simulink model "control_system"  (R2020b)
settings: Solver=FixedStepAuto  StartTime=0.0  StopTime=t_sim  FixedStep=Ts  RelTol=1e-2
values from neighbouring files (symbols this model uses):
  Hp = 10    [main_script.m]
  InitPosX = -2.4980e+03    (= -2498)    [main_script.m]
  InitPosY = -650.5503    [main_script.m]
  InitVelX = V0*cosd(InitYaw)    [main_script.m]
  InitVelY = V0*sind(InitYaw)    [main_script.m]
  InitYaw = 21    [main_script.m]
  lr = 1.592    [main_script.m]
  m = 1625    [main_script.m]
  Ts = 0.1    [main_script.m]
  V0 = 25    [main_script.m]
libraries: neural x856, simulink x1, autolibshared x1, drivingscenarioandsensors x1
(part 21 of 40)

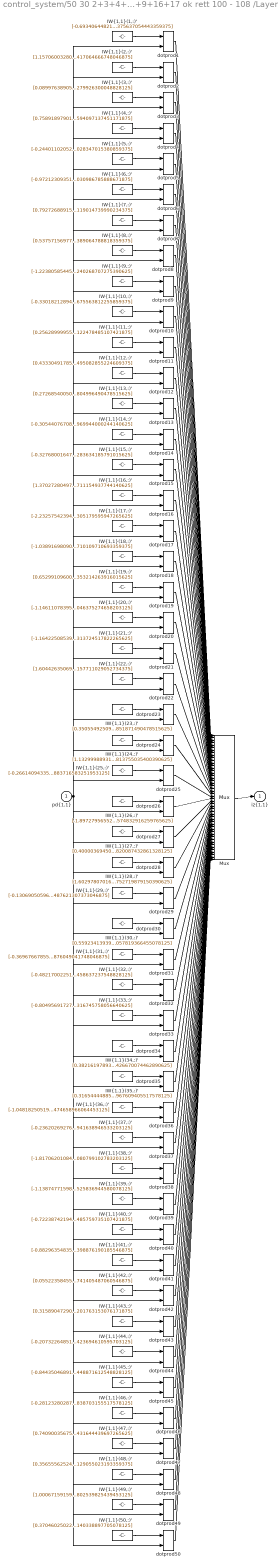
== system control_system/50 30 2+3+4+5+6+7+8+9+16+17 ok rett 100 - 108 /Layer 1/IW{1,1} ==
  "pd{1,1}" : Inport  PortDimensions=9  SampleTime=0.1
      mask Display: e = 0.06;c1 = [120 230 180]/255;c2 = ([120 230 180]+0)/(256+128);c3 = ([120 230 180]+128)/(256+128);patch([0 1 1 0],[0 0 1 1],c1);patch([0 1 1 1-e 1-e 0+e],[0 0 1 1-e 0+e 0+e],c2);patch([0 0 1 1-e 0+e 0+e],[0 1 1 1-e 1-e 0+e],c3);plot([0 1 1 0 0],[0 0 1 1 0]);
  "IW{1,1}(1,:)'" : Constant  Value=[-0.693406448213850001849323234637267887592315673828125;-0.02556518076148506235512058992753736674785614013671875;0.2193186832298505695160173445401596836745738983154296875;1.1520543334356656561823228912544436752796173095703125;-0.40235185759836367136443868730566464364528656005859375;0.90107077061770446402277912056888453662395477294921875;-0.781463922651045361789101661997847259044647216796875;-0.809340341357067227789912067237310111522674560546875;-1.1694920093094791635479623437277041375637054443359375]
      mask Display: e = 0.06;c1 = [120 150 230]/255;c2 = ([120 150 230]+0)/383;c3 = ([120 150 230]+128)/383;patch([0 1 1 0],[0 0 1 1],c1);patch([0 1 1 1-e 1-e 0+e],[0 0 1 1-e 0+e 0+e],c2);patch([0 0 1 1-e 0+e 0+e],[0 1 1 1-e 1-e 0+e],c3);plot([0 1 1 0 0],[0 0 1 1 0]);disp('Weights');
  "IW{1,1}(10,:)'" : Constant  Value=[-0.330182128942806019100686398815014399588108062744140625;0.270379893803715798394904368251445703208446502685546875;-0.97735978725545546996755774671328254044055938720703125;-0.92739473435386254873691314060124568641185760498046875;-0.65365146324644685105198504970758222043514251708984375;2.814218311626336177511120695271529257297515869140625;2.05918257901997403536142883240245282649993896484375;4.88491479731320321633347703027538955211639404296875;-1.173435356109560956383575103245675563812255859375]
      mask Display: e = 0.06;c1 = [120 150 230]/255;c2 = ([120 150 230]+0)/383;c3 = ([120 150 230]+128)/383;patch([0 1 1 0],[0 0 1 1],c1);patch([0 1 1 1-e 1-e 0+e],[0 0 1 1-e 0+e 0+e],c2);patch([0 0 1 1-e 0+e 0+e],[0 1 1 1-e 1-e 0+e],c3);plot([0 1 1 0 0],[0 0 1 1 0]);disp('Weights');
  "IW{1,1}(11,:)'" : Constant  Value=[0.256289999552124891923909899560385383665561676025390625;1.3758001567016198141146787747857160866260528564453125;-0.80612011216949763792172234388999640941619873046875;-0.6585048433570950265902865794487297534942626953125;0.062421786312315645506298977807091432623565196990966796875;0.15111591352368070051426229838398285210132598876953125;-1.301785836379860228362304042093455791473388671875;0.26252656946479202559885379741899669170379638671875;-0.75316510987679929911564613576047122478485107421875]
      mask Display: e = 0.06;c1 = [120 150 230]/255;c2 = ([120 150 230]+0)/383;c3 = ([120 150 230]+128)/383;patch([0 1 1 0],[0 0 1 1],c1);patch([0 1 1 1-e 1-e 0+e],[0 0 1 1-e 0+e 0+e],c2);patch([0 0 1 1-e 0+e 0+e],[0 1 1 1-e 1-e 0+e],c3);plot([0 1 1 0 0],[0 0 1 1 0]);disp('Weights');
  "IW{1,1}(12,:)'" : Constant  Value=[0.43330491785510283353488603097503073513507843017578125;-0.8967160374348315254877661573118530213832855224609375;0.79292956982623585826530643316800706088542938232421875;-0.44560553359943766427164746346534229815006256103515625;0.40491413567924749994375588357797823846340179443359375;-1.8281801022278241219964911579154431819915771484375;-1.794021928142497390723519856692291796207427978515625;1.8148160440597036480170345384976826608180999755859375;0.144981973916790740641857837545103393495082855224609375]
      mask Display: e = 0.06;c1 = [120 150 230]/255;c2 = ([120 150 230]+0)/383;c3 = ([120 150 230]+128)/383;patch([0 1 1 0],[0 0 1 1],c1);patch([0 1 1 1-e 1-e 0+e],[0 0 1 1-e 0+e 0+e],c2);patch([0 0 1 1-e 0+e 0+e],[0 1 1 1-e 1-e 0+e],c3);plot([0 1 1 0 0],[0 0 1 1 0]);disp('Weights');
  "IW{1,1}(13,:)'" : Constant  Value=[0.272685400504414754419002520080539397895336151123046875;0.06475251983479125839071599557428271509706974029541015625;0.0891263580801826271748922181359375827014446258544921875;1.3588154264075875676809346259688027203083038330078125;-0.84834662558519624564468131211469881236553192138671875;-1.7756799833677110456164882634766399860382080078125;-2.108800316675305541735951919690705835819244384765625;2.317421627480893864259314796072430908679962158203125;1.1371762435508954158791539157391525804996490478515625]
      mask Display: e = 0.06;c1 = [120 150 230]/255;c2 = ([120 150 230]+0)/383;c3 = ([120 150 230]+128)/383;patch([0 1 1 0],[0 0 1 1],c1);patch([0 1 1 1-e 1-e 0+e],[0 0 1 1-e 0+e 0+e],c2);patch([0 0 1 1-e 0+e 0+e],[0 1 1 1-e 1-e 0+e],c3);plot([0 1 1 0 0],[0 0 1 1 0]);disp('Weights');
  "IW{1,1}(14,:)'" : Constant  Value=[-0.305440767083966557837726440993719734251499176025390625;1.1031230626814245709965689457021653652191162109375;-0.390168912682526014545913994879811070859432220458984375;1.1610554660892347111911249157856218516826629638671875;-0.37328389762495917114648591450531966984272003173828125;3.2638872617295380251789538306184113025665283203125;0.0203659829001831722827819959320549969561398029327392578125;1.7005610109913560368255502908141352236270904541015625;0.1116923823520036551659728729646303690969944000244140625]
      mask Display: e = 0.06;c1 = [120 150 230]/255;c2 = ([120 150 230]+0)/383;c3 = ([120 150 230]+128)/383;patch([0 1 1 0],[0 0 1 1],c1);patch([0 1 1 1-e 1-e 0+e],[0 0 1 1-e 0+e 0+e],c2);patch([0 0 1 1-e 0+e 0+e],[0 1 1 1-e 1-e 0+e],c3);plot([0 1 1 0 0],[0 0 1 1 0]);disp('Weights');
  "IW{1,1}(15,:)'" : Constant  Value=[-0.32768001647452671409865843088482506573200225830078125;1.172298073364981263466688687913119792938232421875;-0.09920154597840817600751250893154065124690532684326171875;1.4942543874272360415744742567767389118671417236328125;-0.2296467494049061475180906199966557323932647705078125;1.7231626562732567098379377057426609098911285400390625;-0.362349667384589235741287893688422627747058868408203125;1.0058783921240064263002977895666845142841339111328125;0.08797611882380586278973311209483654238283634185791015625]
      mask Display: e = 0.06;c1 = [120 150 230]/255;c2 = ([120 150 230]+0)/383;c3 = ([120 150 230]+128)/383;patch([0 1 1 0],[0 0 1 1],c1);patch([0 1 1 1-e 1-e 0+e],[0 0 1 1-e 0+e 0+e],c2);patch([0 0 1 1-e 0+e 0+e],[0 1 1 1-e 1-e 0+e],c3);plot([0 1 1 0 0],[0 0 1 1 0]);disp('Weights');
  "IW{1,1}(16,:)'" : Constant  Value=[1.37027280497960735061724335537292063236236572265625;0.159288578325931406975968229744466952979564666748046875;1.281773545555778159865667475969530642032623291015625;0.627168919722477458122966709197498857975006103515625;0.53591714582890348506083455504267476499080657958984375;-3.229531631920237177979515763581730425357818603515625;-0.69317652394062323484291709974058903753757476806640625;-2.173242526392685558533912626444362103939056396484375;-0.63066588600048378854268094073631800711154937744140625]
      mask Display: e = 0.06;c1 = [120 150 230]/255;c2 = ([120 150 230]+0)/383;c3 = ([120 150 230]+128)/383;patch([0 1 1 0],[0 0 1 1],c1);patch([0 1 1 1-e 1-e 0+e],[0 0 1 1-e 0+e 0+e],c2);patch([0 0 1 1-e 0+e 0+e],[0 1 1 1-e 1-e 0+e],c3);plot([0 1 1 0 0],[0 0 1 1 0]);disp('Weights');
  "IW{1,1}(17,:)'" : Constant  Value=[-2.232575423946769888061680831015110015869140625;-0.1829004396172365376482815690906136296689510345458984375;1.2677494346707975925170330810942687094211578369140625;-0.87503780474532266708820316125638782978057861328125;0.807021408287351249555285903625190258026123046875;0.23988792042748574573352016159333288669586181640625;1.62198306035521699897117287036962807178497314453125;-0.695423451580790441539647872559726238250732421875;-0.82653776048596316883276813314296305179595947265625]
      mask Display: e = 0.06;c1 = [120 150 230]/255;c2 = ([120 150 230]+0)/383;c3 = ([120 150 230]+128)/383;patch([0 1 1 0],[0 0 1 1],c1);patch([0 1 1 1-e 1-e 0+e],[0 0 1 1-e 0+e 0+e],c2);patch([0 0 1 1-e 0+e 0+e],[0 1 1 1-e 1-e 0+e],c3);plot([0 1 1 0 0],[0 0 1 1 0]);disp('Weights');
  "IW{1,1}(18,:)'" : Constant  Value=[-1.0389169809062208660321857678354717791080474853515625;-1.4630196868647835639620780057157389819622039794921875;0.99642406399851235487830081183346919715404510498046875;-1.170179726715411927528975866152904927730560302734375;-0.51561709388959309219302440396859310567378997802734375;-0.75058668503490622025964285057852976024150848388671875;-0.41577361564194215137746368782245554029941558837890625;0.77508037001214524774894698566640727221965789794921875;-0.748086589386244948940429821959696710109710693359375]
      mask Display: e = 0.06;c1 = [120 150 230]/255;c2 = ([120 150 230]+0)/383;c3 = ([120 150 230]+128)/383;patch([0 1 1 0],[0 0 1 1],c1);patch([0 1 1 1-e 1-e 0+e],[0 0 1 1-e 0+e 0+e],c2);patch([0 0 1 1-e 0+e 0+e],[0 1 1 1-e 1-e 0+e],c3);plot([0 1 1 0 0],[0 0 1 1 0]);disp('Weights');
  "IW{1,1}(19,:)'" : Constant  Value=[0.65299109600750693260806656326167285442352294921875;0.7753435649205380197912518269731663167476654052734375;1.0415876039493869864571706784772686660289764404296875;-0.65848787255995333556057858004351146519184112548828125;1.2322117642516641211614114581607282161712646484375;0.274341649489681593809820014939759857952594757080078125;0.58124655016228865545002690851106308400630950927734375;0.9466010499085590890189223500783555209636688232421875;-0.08066011985930966743385539530208916403353214263916015625]
      mask Display: e = 0.06;c1 = [120 150 230]/255;c2 = ([120 150 230]+0)/383;c3 = ([120 150 230]+128)/383;patch([0 1 1 0],[0 0 1 1],c1);patch([0 1 1 1-e 1-e 0+e],[0 0 1 1-e 0+e 0+e],c2);patch([0 0 1 1-e 0+e 0+e],[0 1 1 1-e 1-e 0+e],c3);plot([0 1 1 0 0],[0 0 1 1 0]);disp('Weights');
  "IW{1,1}(2,:)'" : Constant  Value=[1.1570600328072238038856767161632888019084930419921875;1.903733690245744458735543958027847111225128173828125;-0.389863627068089024785280116702779196202754974365234375;1.746257178047623259686815799796022474765777587890625;0.00989143632890131241364173320107511244714260101318359375;2.7315874512668614215726847760379314422607421875;0.538870059530276446224661412998102605342864990234375;-4.29457801509744996337758493609726428985595703125;1.900650844106816617085087273153476417064666748046875]
      mask Display: e = 0.06;c1 = [120 150 230]/255;c2 = ([120 150 230]+0)/383;c3 = ([120 150 230]+128)/383;patch([0 1 1 0],[0 0 1 1],c1);patch([0 1 1 1-e 1-e 0+e],[0 0 1 1-e 0+e 0+e],c2);patch([0 0 1 1-e 0+e 0+e],[0 1 1 1-e 1-e 0+e],c3);plot([0 1 1 0 0],[0 0 1 1 0]);disp('Weights');
  "IW{1,1}(20,:)'" : Constant  Value=[-1.14611078395096210869041897240094840526580810546875;0.86858056570071473512228976687765680253505706787109375;-1.58842280534746738140938759897835552692413330078125;-0.69376786411447655122941569061367772519588470458984375;0.94198070731023431090278563715401105582714080810546875;-0.94930693977512781156491428191657178103923797607421875;1.1886668013198040672051547517185099422931671142578125;2.44320512274560552867797014187090098857879638671875;0.5842324962664815490853698065620847046375274658203125]
      mask Display: e = 0.06;c1 = [120 150 230]/255;c2 = ([120 150 230]+0)/383;c3 = ([120 150 230]+128)/383;patch([0 1 1 0],[0 0 1 1],c1);patch([0 1 1 1-e 1-e 0+e],[0 0 1 1-e 0+e 0+e],c2);patch([0 0 1 1-e 0+e 0+e],[0 1 1 1-e 1-e 0+e],c3);plot([0 1 1 0 0],[0 0 1 1 0]);disp('Weights');
  "IW{1,1}(21,:)'" : Constant  Value=[-1.1642250853925999454219208928407169878482818603515625;-0.5504932807784437276410471895360387861728668212890625;-1.6869414057329326084300191723741590976715087890625;-0.0028722543247330510791937019376973694306798279285430908203125;0.19023363022934602906133250144193880259990692138671875;-1.20570399485861035060452195466496050357818603515625;-0.1577300337552645093097680728533305227756500244140625;0.2327125275973849494182132957575959153473377227783203125;0.64502475045348950377643859610543586313724517822265625]
      mask Display: e = 0.06;c1 = [120 150 230]/255;c2 = ([120 150 230]+0)/383;c3 = ([120 150 230]+128)/383;patch([0 1 1 0],[0 0 1 1],c1);patch([0 1 1 1-e 1-e 0+e],[0 0 1 1-e 0+e 0+e],c2);patch([0 0 1 1-e 0+e 0+e],[0 1 1 1-e 1-e 0+e],c3);plot([0 1 1 0 0],[0 0 1 1 0]);disp('Weights');
  "IW{1,1}(22,:)'" : Constant  Value=[1.6044263506907328054040817733039148151874542236328125;1.3319671089723590373665729202912189066410064697265625;-1.0851131040152262041686981319799087941646575927734375;2.1355962975134108461361392983235418796539306640625;0.52286735422735119982462492771446704864501953125;-1.645841449463056438418107063625939190387725830078125;1.6714988511291586359419625296141020953655242919921875;-0.1418426114294394080328487461883923970162868499755859375;-1.338735324179674446298804468824528157711029052734375]
      mask Display: e = 0.06;c1 = [120 150 230]/255;c2 = ([120 150 230]+0)/383;c3 = ([120 150 230]+128)/383;patch([0 1 1 0],[0 0 1 1],c1);patch([0 1 1 1-e 1-e 0+e],[0 0 1 1-e 0+e 0+e],c2);patch([0 0 1 1-e 0+e 0+e],[0 1 1 1-e 1-e 0+e],c3);plot([0 1 1 0 0],[0 0 1 1 0]);disp('Weights');
  "IW{1,1}(23,:)'" : Constant  Value=[0.350554925097944225509394300388521514832973480224609375;-1.0931491474881587233625168664730153977870941162109375;0.4203166172719525750522961971000768244266510009765625;-1.394127712399904073237166812759824097156524658203125;-1.3990696404685694087532965568243525922298431396484375;-0.236876967776770808171704629785381257534027099609375;-0.305940597094979171988171628981945104897022247314453125;-0.216334751492993360155736581873497925698757171630859375;0.81177408117963223421753582442761398851871490478515625]
      mask Display: e = 0.06;c1 = [120 150 230]/255;c2 = ([120 150 230]+0)/383;c3 = ([120 150 230]+128)/383;patch([0 1 1 0],[0 0 1 1],c1);patch([0 1 1 1-e 1-e 0+e],[0 0 1 1-e 0+e 0+e],c2);patch([0 0 1 1-e 0+e 0+e],[0 1 1 1-e 1-e 0+e],c3);plot([0 1 1 0 0],[0 0 1 1 0]);disp('Weights');
  "IW{1,1}(24,:)'" : Constant  Value=[1.1329998893150687866437920092721469700336456298828125;-1.4321153177865941774626890037325210869312286376953125;2.591323690879150820620679951389320194721221923828125;1.0806065027108360254715080372989177703857421875;-1.867832138149747578381720813922584056854248046875;1.9590467197986949354771013531717471778392791748046875;1.00821489655478568892021939973346889019012451171875;-0.7955102958743938135199869066127575933933258056640625;-0.59861999316104397284021843006485141813755035400390625]
      mask Display: e = 0.06;c1 = [120 150 230]/255;c2 = ([120 150 230]+0)/383;c3 = ([120 150 230]+128)/383;patch([0 1 1 0],[0 0 1 1],c1);patch([0 1 1 1-e 1-e 0+e],[0 0 1 1-e 0+e 0+e],c2);patch([0 0 1 1-e 0+e 0+e],[0 1 1 1-e 1-e 0+e],c3);plot([0 1 1 0 0],[0 0 1 1 0]);disp('Weights');
  "IW{1,1}(25,:)'" : Constant  Value=[-0.266140943359271575641145091140060685575008392333984375;0.93128971553801409566375468784826807677745819091796875;-0.763023833714053356658268967294134199619293212890625;-1.1174471698171324351989142087404616177082061767578125;0.86052416309833967833498036270611919462680816650390625;1.36946534724734902965792571194469928741455078125;-0.08714593803625887702413166380210896022617816925048828125;0.7130613830161605104507316355011425912380218505859375;0.01361678574539722415270848188129093614406883716583251953125]
      mask Display: e = 0.06;c1 = [120 150 230]/255;c2 = ([120 150 230]+0)/383;c3 = ([120 150 230]+128)/383;patch([0 1 1 0],[0 0 1 1],c1);patch([0 1 1 1-e 1-e 0+e],[0 0 1 1-e 0+e 0+e],c2);patch([0 0 1 1-e 0+e 0+e],[0 1 1 1-e 1-e 0+e],c3);plot([0 1 1 0 0],[0 0 1 1 0]);disp('Weights');
  "IW{1,1}(26,:)'" : Constant  Value=[-1.89727956552465304440602267277427017688751220703125;1.2876139672237514322006290967692621052265167236328125;0.83258954146781138927480014899629168212413787841796875;-2.91139210909474410726716087083332240581512451171875;0.32359731118500378865832090014009736478328704833984375;0.384597586722556117333482461617677472531795501708984375;-0.868477310397982815715067772543989121913909912109375;-0.5317092104185012768624574164277873933315277099609375;1.2926350037718228325189784300164319574832916259765625]
      mask Display: e = 0.06;c1 = [120 150 230]/255;c2 = ([120 150 230]+0)/383;c3 = ([120 150 230]+128)/383;patch([0 1 1 0],[0 0 1 1],c1);patch([0 1 1 1-e 1-e 0+e],[0 0 1 1-e 0+e 0+e],c2);patch([0 0 1 1-e 0+e 0+e],[0 1 1 1-e 1-e 0+e],c3);plot([0 1 1 0 0],[0 0 1 1 0]);disp('Weights');
  "IW{1,1}(27,:)'" : Constant  Value=[0.400003694501827322671516640184563584625720977783203125;-0.85527108082092018204178884843713603913784027099609375;1.4010061502814747935730110839358530938625335693359375;-1.4806639264167633651680944240069948136806488037109375;-0.72477438149454076476985164845245890319347381591796875;1.93831254159486388033428738708607852458953857421875;0.310800466532213548465080066307564266026020050048828125;-2.841585827968680089128383770002983510494232177734375;1.3646232279807606335708669575979001820087432861328125]
      mask Display: e = 0.06;c1 = [120 150 230]/255;c2 = ([120 150 230]+0)/383;c3 = ([120 150 230]+128)/383;patch([0 1 1 0],[0 0 1 1],c1);patch([0 1 1 1-e 1-e 0+e],[0 0 1 1-e 0+e 0+e],c2);patch([0 0 1 1-e 0+e 0+e],[0 1 1 1-e 1-e 0+e],c3);plot([0 1 1 0 0],[0 0 1 1 0]);disp('Weights');
  "IW{1,1}(28,:)'" : Constant  Value=[1.602978070162198065418124315328896045684814453125;-0.3426681801413840045000824829912744462490081787109375;1.529770685331715895927118253894150257110595703125;1.1716836187309633832143163090222515165805816650390625;0.046185804249316120273505248405854217708110809326171875;-0.75021965501111054219762763750622980296611785888671875;1.074021043023239752045583372819237411022186279296875;0.8185220590198494239331239441526122391223907470703125;0.0956170049154911050326433041846030391752719879150390625]
      mask Display: e = 0.06;c1 = [120 150 230]/255;c2 = ([120 150 230]+0)/383;c3 = ([120 150 230]+128)/383;patch([0 1 1 0],[0 0 1 1],c1);patch([0 1 1 1-e 1-e 0+e],[0 0 1 1-e 0+e 0+e],c2);patch([0 0 1 1-e 0+e 0+e],[0 1 1 1-e 1-e 0+e],c3);plot([0 1 1 0 0],[0 0 1 1 0]);disp('Weights');
  "IW{1,1}(29,:)'" : Constant  Value=[-0.1306905059673156010990879849487100727856159210205078125;-0.7876508797924930416201050320523791015148162841796875;-0.51317475975367499163581896937103010714054107666015625;-0.1457425730357558568694997802595025859773159027099609375;-0.70171443760436857939311039444874040782451629638671875;1.27527189707526122930403289501555263996124267578125;0.8890613846162340738743523615994490683078765869140625;0.3216145672896235652160612517036497592926025390625;-1.008127048696333627475496541592292487621307373046875]
      mask Display: e = 0.06;c1 = [120 150 230]/255;c2 = ([120 150 230]+0)/383;c3 = ([120 150 230]+128)/383;patch([0 1 1 0],[0 0 1 1],c1);patch([0 1 1 1-e 1-e 0+e],[0 0 1 1-e 0+e 0+e],c2);patch([0 0 1 1-e 0+e 0+e],[0 1 1 1-e 1-e 0+e],c3);plot([0 1 1 0 0],[0 0 1 1 0]);disp('Weights');
  "IW{1,1}(3,:)'" : Constant  Value=[0.08997638905276246490405611666574259288609027862548828125;0.80681741283027574862529718302539549767971038818359375;0.2250171821611615385894111796005745418369770050048828125;-0.50944131721464402939858473473577760159969329833984375;0.2000247490916989001608072840099339373409748077392578125;1.20314470992705491170227105612866580486297607421875;1.4027922012298004172947685219696722924709320068359375;0.8756386789487733413039904917241074144840240478515625;0.007739900862407400779219290853916390915401279926300048828125]
      mask Display: e = 0.06;c1 = [120 150 230]/255;c2 = ([120 150 230]+0)/383;c3 = ([120 150 230]+128)/383;patch([0 1 1 0],[0 0 1 1],c1);patch([0 1 1 1-e 1-e 0+e],[0 0 1 1-e 0+e 0+e],c2);patch([0 0 1 1-e 0+e 0+e],[0 1 1 1-e 1-e 0+e],c3);plot([0 1 1 0 0],[0 0 1 1 0]);disp('Weights');
  "IW{1,1}(30,:)'" : Constant  Value=[0.55923413939413391116062257424346171319484710693359375;-0.276142396858805538872871920830220915377140045166015625;-0.841140637081708941735769258229993283748626708984375;-1.2799808287890843683243247141945175826549530029296875;0.1619096371925195787522255841395235620439052581787109375;-0.031011122222041880014398174125744844786822795867919921875;-0.67759415806670475479478454872150905430316925048828125;1.1300688296323215809024986810982227325439453125;1.673317340979104006493116685305722057819366455078125]
      mask Display: e = 0.06;c1 = [120 150 230]/255;c2 = ([120 150 230]+0)/383;c3 = ([120 150 230]+128)/383;patch([0 1 1 0],[0 0 1 1],c1);patch([0 1 1 1-e 1-e 0+e],[0 0 1 1-e 0+e 0+e],c2);patch([0 0 1 1-e 0+e 0+e],[0 1 1 1-e 1-e 0+e],c3);plot([0 1 1 0 0],[0 0 1 1 0]);disp('Weights');
  "IW{1,1}(31,:)'" : Constant  Value=[-0.369676678559802074364171176057425327599048614501953125;-0.58159156486953322851007897043018601834774017333984375;1.0786932187140381156353896585642360150814056396484375;0.637537765261984024078856236883439123630523681640625;0.7410181941734403920918339281342923641204833984375;-2.32287606270722779555626402725465595722198486328125;-0.48709727099964605923076987892272882163524627685546875;2.050543368761421181289961168658919632434844970703125;0.48267963789397494434041391286882571876049041748046875]
      mask Display: e = 0.06;c1 = [120 150 230]/255;c2 = ([120 150 230]+0)/383;c3 = ([120 150 230]+128)/383;patch([0 1 1 0],[0 0 1 1],c1);patch([0 1 1 1-e 1-e 0+e],[0 0 1 1-e 0+e 0+e],c2);patch([0 0 1 1-e 0+e 0+e],[0 1 1 1-e 1-e 0+e],c3);plot([0 1 1 0 0],[0 0 1 1 0]);disp('Weights');
  "IW{1,1}(32,:)'" : Constant  Value=[-0.482170022514028573379363251660834066569805145263671875;0.96009191106100166823722474873648025095462799072265625;-0.911853201103436372676469545694999396800994873046875;0.08528072811694854815645072676488780416548252105712890625;1.164210642311785282032587929279543459415435791015625;0.91960001333729401995498164978926070034503936767578125;0.65569530552422905511633643982349894940853118896484375;-1.0546061852062618147130024226498790085315704345703125;-0.63904426441919170986949438884039409458637237548828125]
      mask Display: e = 0.06;c1 = [120 150 230]/255;c2 = ([120 150 230]+0)/383;c3 = ([120 150 230]+128)/383;patch([0 1 1 0],[0 0 1 1],c1);patch([0 1 1 1-e 1-e 0+e],[0 0 1 1-e 0+e 0+e],c2);patch([0 0 1 1-e 0+e 0+e],[0 1 1 1-e 1-e 0+e],c3);plot([0 1 1 0 0],[0 0 1 1 0]);disp('Weights');
  "IW{1,1}(33,:)'" : Constant  Value=[-0.80495691727967433326540458438103087246417999267578125;0.6411180503735127711451013965415768325328826904296875;-1.2023286220364719500963701648288406431674957275390625;-1.599120401012341208257794278324581682682037353515625;-0.0953775174016849580649335393900400958955287933349609375;1.2326435111067846062127273398800753057003021240234375;0.042770745663714880568928577986298478208482265472412109375;1.766417956869078320636390344589017331600189208984375;-0.358630123165513570171469837077893316745758056640625]
      mask Display: e = 0.06;c1 = [120 150 230]/255;c2 = ([120 150 230]+0)/383;c3 = ([120 150 230]+128)/383;patch([0 1 1 0],[0 0 1 1],c1);patch([0 1 1 1-e 1-e 0+e],[0 0 1 1-e 0+e 0+e],c2);patch([0 0 1 1-e 0+e 0+e],[0 1 1 1-e 1-e 0+e],c3);plot([0 1 1 0 0],[0 0 1 1 0]);disp('Weights');
  "IW{1,1}(34,:)'" : Constant  Value=[0.382161978935705970439329348664614371955394744873046875;-0.76302057400596179359553161702933721244335174560546875;0.298250016106143822636198592590517364442348480224609375;-0.70487538233506652485260701723746024072170257568359375;0.0279956842207948232437164648445104830898344516754150390625;-0.68521612708078549758283770643174648284912109375;-0.418788213989499558120854771914309822022914886474609375;-2.727281390156304663463515680632553994655609130859375;-1.277907013729996155149137848638929426670074462890625]
      mask Display: e = 0.06;c1 = [120 150 230]/255;c2 = ([120 150 230]+0)/383;c3 = ([120 150 230]+128)/383;patch([0 1 1 0],[0 0 1 1],c1);patch([0 1 1 1-e 1-e 0+e],[0 0 1 1-e 0+e 0+e],c2);patch([0 0 1 1-e 0+e 0+e],[0 1 1 1-e 1-e 0+e],c3);plot([0 1 1 0 0],[0 0 1 1 0]);disp('Weights');
  "IW{1,1}(35,:)'" : Constant  Value=[0.316544448857396798491237177586299367249011993408203125;0.6155314425673754641366031137295067310333251953125;0.1415964825864601817073662459733895957469940185546875;1.3954169536738867396508112506126053631305694580078125;0.24249578330329757402950008327024988830089569091796875;-1.79231644266071210580548722646199166774749755859375;0.13028961116798576380659824280883185565471649169921875;-0.343855544436020454934777035305160097777843475341796875;-0.75040981724793376361759555948083288967609405517578125]
      mask Display: e = 0.06;c1 = [120 150 230]/255;c2 = ([120 150 230]+0)/383;c3 = ([120 150 230]+128)/383;patch([0 1 1 0],[0 0 1 1],c1);patch([0 1 1 1-e 1-e 0+e],[0 0 1 1-e 0+e 0+e],c2);patch([0 0 1 1-e 0+e 0+e],[0 1 1 1-e 1-e 0+e],c3);plot([0 1 1 0 0],[0 0 1 1 0]);disp('Weights');
  "IW{1,1}(36,:)'" : Constant  Value=[-1.048182505198408609459193030488677322864532470703125;0.5151532139605734528231550939381122589111328125;-2.32440222618064584736430333578027784824371337890625;-0.9589975404242412349020696638035587966442108154296875;-1.161839122224388010096163270645774900913238525390625;-1.8480403874410573639153199110296554863452911376953125;-0.468092609921334001921167100590537302196025848388671875;-2.588322666240973735085617590812034904956817626953125;-0.0293675915841758172764031087353941984474658966064453125]
      mask Display: e = 0.06;c1 = [120 150 230]/255;c2 = ([120 150 230]+0)/383;c3 = ([120 150 230]+128)/383;patch([0 1 1 0],[0 0 1 1],c1);patch([0 1 1 1-e 1-e 0+e],[0 0 1 1-e 0+e 0+e],c2);patch([0 0 1 1-e 0+e 0+e],[0 1 1 1-e 1-e 0+e],c3);plot([0 1 1 0 0],[0 0 1 1 0]);disp('Weights');
  "IW{1,1}(37,:)'" : Constant  Value=[-0.2362026927647044860503200425227987580001354217529296875;-0.78218715596495591579895290124113671481609344482421875;0.8565351137683296922631370762246660888195037841796875;1.4776102515902180822848777097533456981182098388671875;0.453191929204543264564364335456048138439655303955078125;-0.1195925461842739512263733558938838541507720947265625;-0.70882313381148553954602675730711780488491058349609375;-0.480949892098079201385729675166658125817775726318359375;1.5768117638188112739072721524280495941638946533203125]
      mask Display: e = 0.06;c1 = [120 150 230]/255;c2 = ([120 150 230]+0)/383;c3 = ([120 150 230]+128)/383;patch([0 1 1 0],[0 0 1 1],c1);patch([0 1 1 1-e 1-e 0+e],[0 0 1 1-e 0+e 0+e],c2);patch([0 0 1 1-e 0+e 0+e],[0 1 1 1-e 1-e 0+e],c3);plot([0 1 1 0 0],[0 0 1 1 0]);disp('Weights');
  "IW{1,1}(38,:)'" : Constant  Value=[-1.8170620108458077623936333111487329006195068359375;-0.836309493935304626432980512618087232112884521484375;0.347037295405833778882964679723954759538173675537109375;-1.1257424830385394098897222647792659699916839599609375;-1.5102367218942529536462870964896865189075469970703125;-1.16258945977454342113333041197620332241058349609375;0.040529601691721740819307484571254462935030460357666015625;-1.762905379354144930204029151354916393756866455078125;1.369967279907751578349461851757951080799102783203125]
      mask Display: e = 0.06;c1 = [120 150 230]/255;c2 = ([120 150 230]+0)/383;c3 = ([120 150 230]+128)/383;patch([0 1 1 0],[0 0 1 1],c1);patch([0 1 1 1-e 1-e 0+e],[0 0 1 1-e 0+e 0+e],c2);patch([0 0 1 1-e 0+e 0+e],[0 1 1 1-e 1-e 0+e],c3);plot([0 1 1 0 0],[0 0 1 1 0]);disp('Weights');
  "IW{1,1}(39,:)'" : Constant  Value=[-1.1387477159820329486450418698950670659542083740234375;0.12329538400851185186990477404833654873073101043701171875;-1.2901694683843327737804429489187896251678466796875;0.482497177772101382142722059143125079572200775146484375;-0.46053829469796248030633023518021218478679656982421875;0.8066115310647157254919648039503954350948333740234375;0.362412929683291640259312771377153694629669189453125;-0.3922292711960551070404790152679197490215301513671875;-0.9901181825802745084530442909453995525836944580078125]
      mask Display: e = 0.06;c1 = [120 150 230]/255;c2 = ([120 150 230]+0)/383;c3 = ([120 150 230]+128)/383;patch([0 1 1 0],[0 0 1 1],c1);patch([0 1 1 1-e 1-e 0+e],[0 0 1 1-e 0+e 0+e],c2);patch([0 0 1 1-e 0+e 0+e],[0 1 1 1-e 1-e 0+e],c3);plot([0 1 1 0 0],[0 0 1 1 0]);disp('Weights');
  "IW{1,1}(4,:)'" : Constant  Value=[0.75891897901968963235930232258397154510021209716796875;1.0908727108738067723692211075103841722011566162109375;0.175572791832671881717686801493982784450054168701171875;0.282146094678743131201059668455854989588260650634765625;-0.410839866592748903517673397800535894930362701416015625;-3.03464107783192194034427302540279924869537353515625;-0.42858137539071849975158556844689883291721343994140625;-0.487092370157764964488933401298709213733673095703125;0.31852922151936169381514218912343494594097137451171875]
      mask Display: e = 0.06;c1 = [120 150 230]/255;c2 = ([120 150 230]+0)/383;c3 = ([120 150 230]+128)/383;patch([0 1 1 0],[0 0 1 1],c1);patch([0 1 1 1-e 1-e 0+e],[0 0 1 1-e 0+e 0+e],c2);patch([0 0 1 1-e 0+e 0+e],[0 1 1 1-e 1-e 0+e],c3);plot([0 1 1 0 0],[0 0 1 1 0]);disp('Weights');
  "IW{1,1}(40,:)'" : Constant  Value=[-0.7223874219432262488993501392542384564876556396484375;0.15416300451654663117295740448753349483013153076171875;0.5813294583854677899381613315199501812458038330078125;0.98923721451935542336997286838595755398273468017578125;-0.9903292416109705786908534719259478151798248291015625;-0.528718596441362986837475546053610742092132568359375;0.871554716413495800253485867870040237903594970703125;-1.2409986381583573145093168932362459599971771240234375;0.971169333727583961035634274594485759735107421875]
      mask Display: e = 0.06;c1 = [120 150 230]/255;c2 = ([120 150 230]+0)/383;c3 = ([120 150 230]+128)/383;patch([0 1 1 0],[0 0 1 1],c1);patch([0 1 1 1-e 1-e 0+e],[0 0 1 1-e 0+e 0+e],c2);patch([0 0 1 1-e 0+e 0+e],[0 1 1 1-e 1-e 0+e],c3);plot([0 1 1 0 0],[0 0 1 1 0]);disp('Weights');
  "IW{1,1}(41,:)'" : Constant  Value=[-0.882963548351868521280039203702472150325775146484375;0.91675878904890295562069013612926937639713287353515625;1.011914513744740506950847702682949602603912353515625;-1.574378303396426925786499850801192224025726318359375;-1.197888213693703018947189775644801557064056396484375;0.100287539056347407839808738572173751890659332275390625;0.53232743683504912812765041962848044931888580322265625;0.378933387288537926185227888709050603210926055908203125;1.06883057548883453335974991205148398876190185546875]
      mask Display: e = 0.06;c1 = [120 150 230]/255;c2 = ([120 150 230]+0)/383;c3 = ([120 150 230]+128)/383;patch([0 1 1 0],[0 0 1 1],c1);patch([0 1 1 1-e 1-e 0+e],[0 0 1 1-e 0+e 0+e],c2);patch([0 0 1 1-e 0+e 0+e],[0 1 1 1-e 1-e 0+e],c3);plot([0 1 1 0 0],[0 0 1 1 0]);disp('Weights');
  "IW{1,1}(42,:)'" : Constant  Value=[0.0552235845579313877617977368572610430419445037841796875;0.86593509061196682896621723557473160326480865478515625;-1.6191474070289222364493753048009239137172698974609375;-0.41717605629963916413771585212089121341705322265625;1.40814378549649887872874387539923191070556640625;0.041060184405020801190477897080199909396469593048095703125;0.63687594197354713276837401281227357685565948486328125;-1.5333877445710257791944286509533412754535675048828125;0.5832473178880188680039964310708455741405487060546875]
      mask Display: e = 0.06;c1 = [120 150 230]/255;c2 = ([120 150 230]+0)/383;c3 = ([120 150 230]+128)/383;patch([0 1 1 0],[0 0 1 1],c1);patch([0 1 1 1-e 1-e 0+e],[0 0 1 1-e 0+e 0+e],c2);patch([0 0 1 1-e 0+e 0+e],[0 1 1 1-e 1-e 0+e],c3);plot([0 1 1 0 0],[0 0 1 1 0]);disp('Weights');
  "IW{1,1}(43,:)'" : Constant  Value=[0.315890472905115238244633246722514741122722625732421875;-0.8771203406882805975186556679545901715755462646484375;-0.36208714197739400031395007317769341170787811279296875;-0.685894407660199600940131858806125819683074951171875;-0.90178038620316913753782728235819377005100250244140625;-0.846092021704275776272652365150861442089080810546875;-0.260067493991034126565864426083862781524658203125;-0.8606971664539724287124045076780021190643310546875;0.98339367262981525197318433129112236201763153076171875]
      mask Display: e = 0.06;c1 = [120 150 230]/255;c2 = ([120 150 230]+0)/383;c3 = ([120 150 230]+128)/383;patch([0 1 1 0],[0 0 1 1],c1);patch([0 1 1 1-e 1-e 0+e],[0 0 1 1-e 0+e 0+e],c2);patch([0 0 1 1-e 0+e 0+e],[0 1 1 1-e 1-e 0+e],c3);plot([0 1 1 0 0],[0 0 1 1 0]);disp('Weights');
  "IW{1,1}(44,:)'" : Constant  Value=[-0.207322648518014240881512932901387102901935577392578125;1.0633974658595064521904305365751497447490692138671875;-0.5382910098955731026393323190859518945217132568359375;0.10413169816160509906222131348840775899589061737060546875;0.419802792782568767737672033035778440535068511962890625;0.56162037806451559074361057355417869985103607177734375;0.07006108163071776695485226582604809664189815521240234375;-1.0330617265353210232348146746517159044742584228515625;-1.312650593385850772421008514356799423694610595703125]
      mask Display: e = 0.06;c1 = [120 150 230]/255;c2 = ([120 150 230]+0)/383;c3 = ([120 150 230]+128)/383;patch([0 1 1 0],[0 0 1 1],c1);patch([0 1 1 1-e 1-e 0+e],[0 0 1 1-e 0+e 0+e],c2);patch([0 0 1 1-e 0+e 0+e],[0 1 1 1-e 1-e 0+e],c3);plot([0 1 1 0 0],[0 0 1 1 0]);disp('Weights');
  "IW{1,1}(45,:)'" : Constant  Value=[-0.84435046891182830020028404760523699223995208740234375;1.0482276873537010875025998757337220013141632080078125;0.9442997627094886770038328904774971306324005126953125;0.302979639012098289629904002140392549335956573486328125;0.1302338684863636186772595237925997935235500335693359375;0.32870165743802004509888092798064462840557098388671875;-0.8024789792089668249985834336257539689540863037109375;-0.71114351671465370063884847695589996874332427978515625;-0.62380436905905256583793061508913524448871612548828125]
      mask Display: e = 0.06;c1 = [120 150 230]/255;c2 = ([120 150 230]+0)/383;c3 = ([120 150 230]+128)/383;patch([0 1 1 0],[0 0 1 1],c1);patch([0 1 1 1-e 1-e 0+e],[0 0 1 1-e 0+e 0+e],c2);patch([0 0 1 1-e 0+e 0+e],[0 1 1 1-e 1-e 0+e],c3);plot([0 1 1 0 0],[0 0 1 1 0]);disp('Weights');
  "IW{1,1}(46,:)'" : Constant  Value=[-0.281232802871846043757386723882518708705902099609375;0.87424712198429055387549624356324784457683563232421875;-1.3778829356479196377449625288136303424835205078125;-0.780221340687571540684075444005429744720458984375;1.219842642544281208216716549941338598728179931640625;0.7050205886415679135126310939085669815540313720703125;-0.43121835582297318723021817277185618877410888671875;0.1408004974160800559790374109070398844778537750244140625;0.007699606648294885120897834696052086655981838703155517578125]
      mask Display: e = 0.06;c1 = [120 150 230]/255;c2 = ([120 150 230]+0)/383;c3 = ([120 150 230]+128)/383;patch([0 1 1 0],[0 0 1 1],c1);patch([0 1 1 1-e 1-e 0+e],[0 0 1 1-e 0+e 0+e],c2);patch([0 0 1 1-e 0+e 0+e],[0 1 1 1-e 1-e 0+e],c3);plot([0 1 1 0 0],[0 0 1 1 0]);disp('Weights');
  "IW{1,1}(47,:)'" : Constant  Value=[0.74090035675614351884377128953929059207439422607421875;-0.1963066385750354692074637341647758148610591888427734375;0.099354390568328287969279699609614908695220947265625;-0.88848868625771337814711614555562846362590789794921875;0.407218011039563287933873425572528503835201263427734375;-1.4108429642830195849256824658368714153766632080078125;-0.0690369977490646047346700697744381614029407501220703125;0.10921138485657154448826844372888444922864437103271484375;-1.2294240135385428036585153677151538431644439697265625]
      mask Display: e = 0.06;c1 = [120 150 230]/255;c2 = ([120 150 230]+0)/383;c3 = ([120 150 230]+128)/383;patch([0 1 1 0],[0 0 1 1],c1);patch([0 1 1 1-e 1-e 0+e],[0 0 1 1-e 0+e 0+e],c2);patch([0 0 1 1-e 0+e 0+e],[0 1 1 1-e 1-e 0+e],c3);plot([0 1 1 0 0],[0 0 1 1 0]);disp('Weights');
  "IW{1,1}(48,:)'" : Constant  Value=[0.3565556252466415276813904711161740124225616455078125;1.1230800437348704701179258336196653544902801513671875;-1.101252085483165554791185059002600610256195068359375;0.1824000649953292640947921654515084810554981231689453125;-0.70473688538656131807869087424478493630886077880859375;-1.0628344260220654593496192319435067474842071533203125;0.88925987521902494226111457464867271482944488525390625;-0.0143711829375529932806276889323271461762487888336181640625;-0.60994083293363754449956104508601129055023193359375]
      mask Display: e = 0.06;c1 = [120 150 230]/255;c2 = ([120 150 230]+0)/383;c3 = ([120 150 230]+128)/383;patch([0 1 1 0],[0 0 1 1],c1);patch([0 1 1 1-e 1-e 0+e],[0 0 1 1-e 0+e 0+e],c2);patch([0 0 1 1-e 0+e 0+e],[0 1 1 1-e 1-e 0+e],c3);plot([0 1 1 0 0],[0 0 1 1 0]);disp('Weights');
  "IW{1,1}(49,:)'" : Constant  Value=[1.0006715915915600501051585524692200124263763427734375;0.67449719974324617854932739646756090223789215087890625;-0.2486319798768005517874968290925608016550540924072265625;0.79586457974658575409421246149577200412750244140625;1.194184895286099834521564844180829823017120361328125;0.1080907671364091104937443788003292866051197052001953125;-0.0099938103556189324117031702598978881724178791046142578125;1.0706456432337236872598396075773052871227264404296875;1.1483539672738249937111731924233026802539825439453125]
      mask Display: e = 0.06;c1 = [120 150 230]/255;c2 = ([120 150 230]+0)/383;c3 = ([120 150 230]+128)/383;patch([0 1 1 0],[0 0 1 1],c1);patch([0 1 1 1-e 1-e 0+e],[0 0 1 1-e 0+e 0+e],c2);patch([0 0 1 1-e 0+e 0+e],[0 1 1 1-e 1-e 0+e],c3);plot([0 1 1 0 0],[0 0 1 1 0]);disp('Weights');
  "IW{1,1}(5,:)'" : Constant  Value=[-0.2440110205213656957567991412361152470111846923828125;-1.1118649633055366354739135203999467194080352783203125;0.0305537306978848725858011192713092896156013011932373046875;0.60990936599379430571588045495445840060710906982421875;1.1011154013702466603064067385275848209857940673828125;-0.68761892786242240216409982167533598840236663818359375;-0.21127451839044464332317829757812432944774627685546875;0.61383190906246232199094947645789943635463714599609375;-0.91900525903316532261300153550109826028347015380859375]
      mask Display: e = 0.06;c1 = [120 150 230]/255;c2 = ([120 150 230]+0)/383;c3 = ([120 150 230]+128)/383;patch([0 1 1 0],[0 0 1 1],c1);patch([0 1 1 1-e 1-e 0+e],[0 0 1 1-e 0+e 0+e],c2);patch([0 0 1 1-e 0+e 0+e],[0 1 1 1-e 1-e 0+e],c3);plot([0 1 1 0 0],[0 0 1 1 0]);disp('Weights');
  "IW{1,1}(50,:)'" : Constant  Value=[0.370460250225562059966932793031446635723114013671875;-1.1041072265145375208561517865746282041072845458984375;0.7156606806565617429072290178737603127956390380859375;0.35444152424409647306191573079559020698070526123046875;0.40298401322406818270138728621532209217548370361328125;1.8335591910250188529829529215930961072444915771484375;-0.138757828064884625174357779542333446443080902099609375;-0.896201029056029607744449094752781093120574951171875;1.26510160276534566747841381584294140338897705078125]
      mask Display: e = 0.06;c1 = [120 150 230]/255;c2 = ([120 150 230]+0)/383;c3 = ([120 150 230]+128)/383;patch([0 1 1 0],[0 0 1 1],c1);patch([0 1 1 1-e 1-e 0+e],[0 0 1 1-e 0+e 0+e],c2);patch([0 0 1 1-e 0+e 0+e],[0 1 1 1-e 1-e 0+e],c3);plot([0 1 1 0 0],[0 0 1 1 0]);disp('Weights');
  "IW{1,1}(6,:)'" : Constant  Value=[-0.97212309351691661429839541597175411880016326904296875;-1.1952763158866381854039673271472565829753875732421875;1.4429456276529302183320169206126593053340911865234375;0.0698389575047022870268875749388826079666614532470703125;-0.136427872157859841895088948149350471794605255126953125;0.71726301695449412587635151794529519975185394287109375;0.1073461498140137193590959441280574537813663482666015625;1.55866863181723136477785374154336750507354736328125;0.58637426424349115006151578199933283030986785888671875]
      mask Display: e = 0.06;c1 = [120 150 230]/255;c2 = ([120 150 230]+0)/383;c3 = ([120 150 230]+128)/383;patch([0 1 1 0],[0 0 1 1],c1);patch([0 1 1 1-e 1-e 0+e],[0 0 1 1-e 0+e 0+e],c2);patch([0 0 1 1-e 0+e 0+e],[0 1 1 1-e 1-e 0+e],c3);plot([0 1 1 0 0],[0 0 1 1 0]);disp('Weights');
  "IW{1,1}(7,:)'" : Constant  Value=[0.79272688915705658008192813213099725544452667236328125;0.817095889661777707857481800601817667484283447265625;-2.042416437605813595013160011149011552333831787109375;-1.5537381213735683704868506538332439959049224853515625;0.303151890975864091171132486124406568706035614013671875;-3.488978582295439334615139159723185002803802490234375;1.4383802695832292872779589743004180490970611572265625;0.70268685026520383285486559543642215430736541748046875;-0.154221259174403380054485523942275904119014739990234375]
      mask Display: e = 0.06;c1 = [120 150 230]/255;c2 = ([120 150 230]+0)/383;c3 = ([120 150 230]+128)/383;patch([0 1 1 0],[0 0 1 1],c1);patch([0 1 1 1-e 1-e 0+e],[0 0 1 1-e 0+e 0+e],c2);patch([0 0 1 1-e 0+e 0+e],[0 1 1 1-e 1-e 0+e],c3);plot([0 1 1 0 0],[0 0 1 1 0]);disp('Weights');
  "IW{1,1}(8,:)'" : Constant  Value=[0.5375715697741096921191683577490039169788360595703125;-0.56098881511250286990843960666097700595855712890625;0.441448539777194337574428573134355247020721435546875;0.82255954334839087582764705075533129274845123291015625;0.07966549549353231507442529846230172552168369293212890625;1.1067926075936493912621472190949134528636932373046875;-1.4087819066734070805324563480098731815814971923828125;-1.4790826708339237516298680930049158632755279541015625;-0.560733482206385414059468530467711389064788818359375]
      mask Display: e = 0.06;c1 = [120 150 230]/255;c2 = ([120 150 230]+0)/383;c3 = ([120 150 230]+128)/383;patch([0 1 1 0],[0 0 1 1],c1);patch([0 1 1 1-e 1-e 0+e],[0 0 1 1-e 0+e 0+e],c2);patch([0 0 1 1-e 0+e 0+e],[0 1 1 1-e 1-e 0+e],c3);plot([0 1 1 0 0],[0 0 1 1 0]);disp('Weights');
  "IW{1,1}(9,:)'" : Constant  Value=[-1.2238058544529426541203065426088869571685791015625;1.669110275596514814111515079275704920291900634765625;0.63863597992205189957104494169470854103565216064453125;-0.87394034853449198418928745013545267283916473388671875;0.84418070402385858574945132204447872936725616455078125;-0.2040911364399825289606127398656099103391170501708984375;-0.739049415296234801786567913950420916080474853515625;-0.1708527803337433204067252745517180301249027252197265625;-2.009738779404381947557567400508560240268707275390625]
      mask Display: e = 0.06;c1 = [120 150 230]/255;c2 = ([120 150 230]+0)/383;c3 = ([120 150 230]+128)/383;patch([0 1 1 0],[0 0 1 1],c1);patch([0 1 1 1-e 1-e 0+e],[0 0 1 1-e 0+e 0+e],c2);patch([0 0 1 1-e 0+e 0+e],[0 1 1 1-e 1-e 0+e],c3);plot([0 1 1 0 0],[0 0 1 1 0]);disp('Weights');
  Mux : Mux  Inputs=50
      mask Display: e = 0.06;c1 = [120 150 230]/255;c2 = ([120 150 230]+0)/383;c3 = ([120 150 230]+128)/383;patch([0 1 1 0],[0 0 1 1],c1);patch([0 1 1 1-e 1-e 0+e],[0 0 1 1-e 0+e 0+e],c2);patch([0 0 1 1-e 0+e 0+e],[0 1 1 1-e 1-e 0+e],c3);plot([0 1 1 0 0],[0 0 1 1 0]);disp('Mux');
  dotprod{1..50} (50 alike) : neural/Weight Functions/dotprod
  "iz{1,1}" : Outport
      mask Display: e = 0.06;c1 = [120 230 180]/255;c2 = ([120 230 180]+0)/(256+128);c3 = ([120 230 180]+128)/(256+128);patch([0 1 1 0],[0 0 1 1],c1);patch([0 1 1 1-e 1-e 0+e],[0 0 1 1-e 0+e 0+e],c2);patch([0 0 1 1-e 0+e 0+e],[0 1 1 1-e 1-e 0+e],c3);plot([0 1 1 0 0],[0 0 1 1 0]);
  wires:
  "IW{1,1}(1,:)'"/1 -> dotprod1/1
  "pd{1,1}"/1 -> dotprod1/2, dotprod2/2, dotprod3/2, dotprod4/2, dotprod5/2, dotprod6/2, dotprod7/2, dotprod8/2, dotprod9/2, dotprod10/2, dotprod11/2, dotprod12/2, dotprod13/2, dotprod14/2, dotprod15/2, dotprod16/2, dotprod17/2, dotprod18/2, dotprod19/2, dotprod20/2, dotprod21/2, dotprod22/2, dotprod23/2, dotprod24/2, dotprod25/2, dotprod26/2, dotprod27/2, dotprod28/2, dotprod29/2, dotprod30/2, dotprod31/2, dotprod32/2, dotprod33/2, dotprod34/2, dotprod35/2, dotprod36/2, dotprod37/2, dotprod38/2, dotprod39/2, dotprod40/2, dotprod41/2, dotprod42/2, dotprod43/2, dotprod44/2, dotprod45/2, dotprod46/2, dotprod47/2, dotprod48/2, dotprod49/2, dotprod50/2
  dotprod1/1 -> Mux/1
  "IW{1,1}(2,:)'"/1 -> dotprod2/1
  dotprod2/1 -> Mux/2
  "IW{1,1}(3,:)'"/1 -> dotprod3/1
  dotprod3/1 -> Mux/3
  "IW{1,1}(4,:)'"/1 -> dotprod4/1
  dotprod4/1 -> Mux/4
  "IW{1,1}(5,:)'"/1 -> dotprod5/1
  dotprod5/1 -> Mux/5
  "IW{1,1}(6,:)'"/1 -> dotprod6/1
  dotprod6/1 -> Mux/6
  "IW{1,1}(7,:)'"/1 -> dotprod7/1
  dotprod7/1 -> Mux/7
  "IW{1,1}(8,:)'"/1 -> dotprod8/1
  dotprod8/1 -> Mux/8
  "IW{1,1}(9,:)'"/1 -> dotprod9/1
  dotprod9/1 -> Mux/9
  "IW{1,1}(10,:)'"/1 -> dotprod10/1
  dotprod10/1 -> Mux/10
  "IW{1,1}(11,:)'"/1 -> dotprod11/1
  dotprod11/1 -> Mux/11
  "IW{1,1}(12,:)'"/1 -> dotprod12/1
  dotprod12/1 -> Mux/12
  "IW{1,1}(13,:)'"/1 -> dotprod13/1
  dotprod13/1 -> Mux/13
  "IW{1,1}(14,:)'"/1 -> dotprod14/1
  dotprod14/1 -> Mux/14
  "IW{1,1}(15,:)'"/1 -> dotprod15/1
  dotprod15/1 -> Mux/15
  "IW{1,1}(16,:)'"/1 -> dotprod16/1
  dotprod16/1 -> Mux/16
  "IW{1,1}(17,:)'"/1 -> dotprod17/1
  dotprod17/1 -> Mux/17
  "IW{1,1}(18,:)'"/1 -> dotprod18/1
  dotprod18/1 -> Mux/18
  "IW{1,1}(19,:)'"/1 -> dotprod19/1
  dotprod19/1 -> Mux/19
  "IW{1,1}(20,:)'"/1 -> dotprod20/1
  dotprod20/1 -> Mux/20
  "IW{1,1}(21,:)'"/1 -> dotprod21/1
  dotprod21/1 -> Mux/21
  "IW{1,1}(22,:)'"/1 -> dotprod22/1
  dotprod22/1 -> Mux/22
  "IW{1,1}(23,:)'"/1 -> dotprod23/1
  dotprod23/1 -> Mux/23
  "IW{1,1}(24,:)'"/1 -> dotprod24/1
  dotprod24/1 -> Mux/24
  "IW{1,1}(25,:)'"/1 -> dotprod25/1
  dotprod25/1 -> Mux/25
  "IW{1,1}(26,:)'"/1 -> dotprod26/1
  dotprod26/1 -> Mux/26
  "IW{1,1}(27,:)'"/1 -> dotprod27/1
  dotprod27/1 -> Mux/27
  "IW{1,1}(28,:)'"/1 -> dotprod28/1
  dotprod28/1 -> Mux/28
  "IW{1,1}(29,:)'"/1 -> dotprod29/1
  dotprod29/1 -> Mux/29
  "IW{1,1}(30,:)'"/1 -> dotprod30/1
  dotprod30/1 -> Mux/30
  "IW{1,1}(31,:)'"/1 -> dotprod31/1
  dotprod31/1 -> Mux/31
  "IW{1,1}(32,:)'"/1 -> dotprod32/1
  dotprod32/1 -> Mux/32
  "IW{1,1}(33,:)'"/1 -> dotprod33/1
  dotprod33/1 -> Mux/33
  "IW{1,1}(34,:)'"/1 -> dotprod34/1
  dotprod34/1 -> Mux/34
  "IW{1,1}(35,:)'"/1 -> dotprod35/1
  dotprod35/1 -> Mux/35
  "IW{1,1}(36,:)'"/1 -> dotprod36/1
  dotprod36/1 -> Mux/36
  "IW{1,1}(37,:)'"/1 -> dotprod37/1
  dotprod37/1 -> Mux/37
  "IW{1,1}(38,:)'"/1 -> dotprod38/1
  dotprod38/1 -> Mux/38
  "IW{1,1}(39,:)'"/1 -> dotprod39/1
  dotprod39/1 -> Mux/39
  "IW{1,1}(40,:)'"/1 -> dotprod40/1
  dotprod40/1 -> Mux/40
  "IW{1,1}(41,:)'"/1 -> dotprod41/1
  dotprod41/1 -> Mux/41
  "IW{1,1}(42,:)'"/1 -> dotprod42/1
  dotprod42/1 -> Mux/42
  "IW{1,1}(43,:)'"/1 -> dotprod43/1
  dotprod43/1 -> Mux/43
  "IW{1,1}(44,:)'"/1 -> dotprod44/1
  dotprod44/1 -> Mux/44
  "IW{1,1}(45,:)'"/1 -> dotprod45/1
  dotprod45/1 -> Mux/45
  "IW{1,1}(46,:)'"/1 -> dotprod46/1
  dotprod46/1 -> Mux/46
  "IW{1,1}(47,:)'"/1 -> dotprod47/1
  dotprod47/1 -> Mux/47
  "IW{1,1}(48,:)'"/1 -> dotprod48/1
  dotprod48/1 -> Mux/48
  "IW{1,1}(49,:)'"/1 -> dotprod49/1
  dotprod49/1 -> Mux/49
  "IW{1,1}(50,:)'"/1 -> dotprod50/1
  dotprod50/1 -> Mux/50
  Mux/1 -> "iz{1,1}"/1

== system control_system/50 30 2+3+4+5+6+7+8+9+16+17 ok rett 100 - 108 /Layer 2/Delays 1 ==
  "p{2}" : Inport  PortDimensions=50  SampleTime=0.1
      mask Display: e = 0.06;c1 = [120 230 180]/255;c2 = ([120 230 180]+0)/(256+128);c3 = ([120 230 180]+128)/(256+128);patch([0 1 1 0],[0 0 1 1],c1);patch([0 1 1 1-e 1-e 0+e],[0 0 1 1-e 0+e 0+e],c2);patch([0 0 1 1-e 0+e 0+e],[0 1 1 1-e 1-e 0+e],c3);plot([0 1 1 0 0],[0 0 1 1 0]);
  mux : Mux  Inputs=1
      mask Display: e = 0.06;c1 = [120 150 230]/255;c2 = ([120 150 230]+0)/383;c3 = ([120 150 230]+128)/383;patch([0 1 1 0],[0 0 1 1],c1);patch([0 1 1 1-e 1-e 0+e],[0 0 1 1-e 0+e 0+e],c2);patch([0 0 1 1-e 0+e 0+e],[0 1 1 1-e 1-e 0+e],c3);plot([0 1 1 0 0],[0 0 1 1 0]);disp('Mux')
  "pd{2,1}" : Outport
      mask Display: e = 0.06;c1 = [120 230 180]/255;c2 = ([120 230 180]+0)/(256+128);c3 = ([120 230 180]+128)/(256+128);patch([0 1 1 0],[0 0 1 1],c1);patch([0 1 1 1-e 1-e 0+e],[0 0 1 1-e 0+e 0+e],c2);patch([0 0 1 1-e 0+e 0+e],[0 1 1 1-e 1-e 0+e],c3);plot([0 1 1 0 0],[0 0 1 1 0]);
  wires:
  "p{2}"/1 -> mux/1
  mux/1 -> "pd{2,1}"/1
